simulink model "vMCU_model"  (R2024b)
settings: Solver=FixedStepAuto  StartTime=0.0  StopTime=0.15  FixedStep=125e-9  RelTol=1e-3
undefined symbols (not defined in the file): den, num
settings Model: Creator=matti  LastModifiedBy=Andrei
settings SolverCC: AlgebraicLoopSolver=TrustRegion
settings DebuggingCC: UnconnectedInputMsg=warning  UnconnectedOutputMsg=warning  UnconnectedLineMsg=warning
settings ModelReferenceCC: EnableRefExpFcnMdlSchedulingChecks=on
settings RTWCC: GPUComputeCapability=3.5

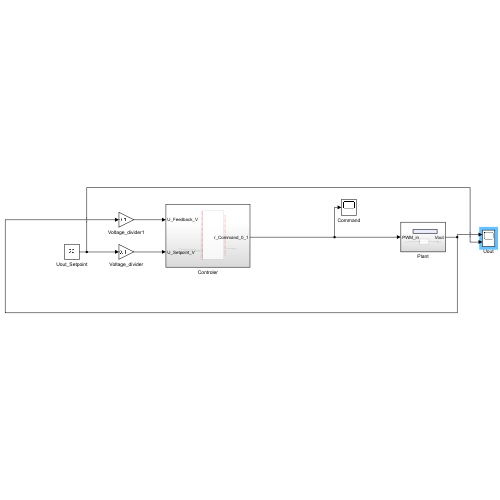
[thumbnail: Simulink's stored preview of the top-level diagram]
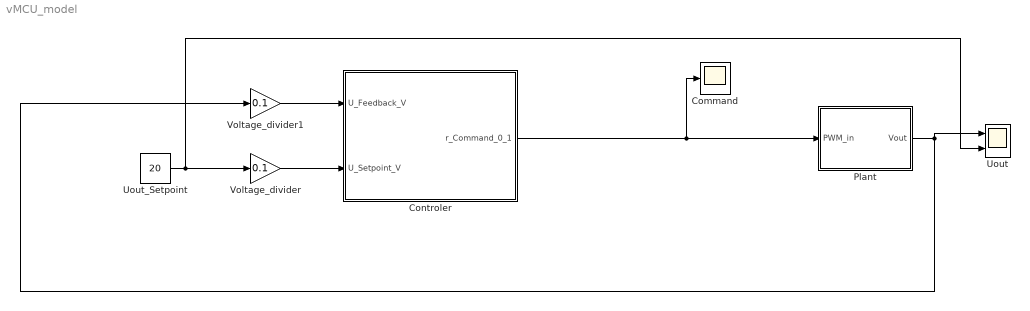
== system vMCU_model ==
  Command : Scope
  Controler : Subsystem
  Plant : Subsystem
  Uout : Scope  NumInputPorts=2
  Uout_Setpoint : Constant  Value=20
  Voltage_divider : Gain  Gain=0.1
  Voltage_divider1 : Gain  Gain=0.1
  wires:
  Voltage_divider1/1 -> Controler/1(U_Feedback_V)
  Uout_Setpoint/1 -> Uout/2, Voltage_divider/1
  Controler/1(r_Command_0_1) -> Plant/1(PWM_in), Command/1
  Plant/1(Vout) -> Voltage_divider1/1, Uout/1
  Voltage_divider/1 -> Controler/2(U_Setpoint_V)

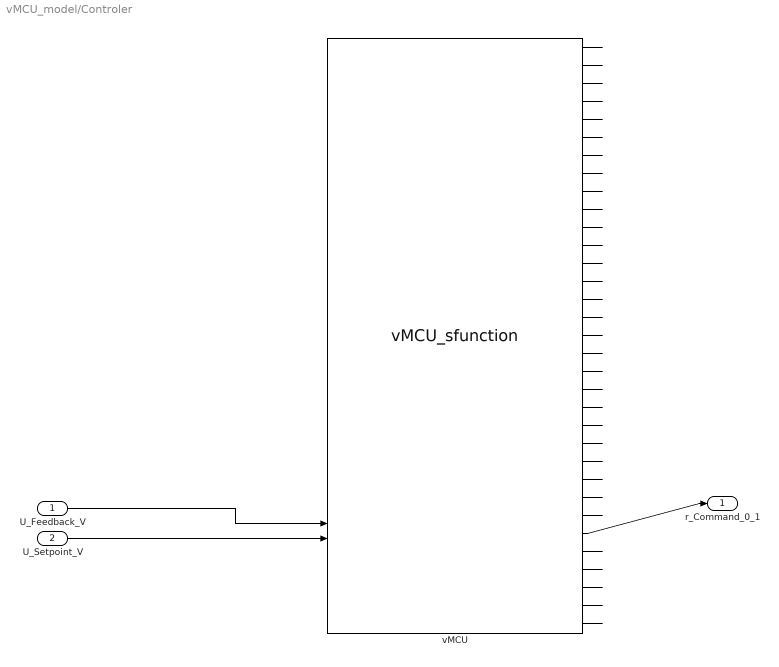
== system vMCU_model/Controler ==
  U_Feedback_V : Inport
  U_Setpoint_V : Inport  Port=2
  vMCU : S-Function  FunctionName=vMCU_sfunction  SFunctionDeploymentMode=off  EnableBusSupport=off
      mask Display:
      | port_label('output', 1, 'vPA0_O_D')
      | port_label('output', 2, 'vPA1_O_D')
      | port_label('output', 3, 'vPA2_O_D')
      | port_label('output', 4, 'vPA3_O_D')
      | port_label('output', 5, 'vPA4_O_D')
      | port_label('output', 6, 'vPA5_O_D')
      | port_label('output', 7, 'vPA6_O_D')
      | port_label('output', 8, 'vPA7_O_D')
      | port_label('output', 9, 'vPB0_O_D')
      | port_label('output', 10, 'vPB1_O_D')
      | port_label('output', 11, 'vPB2_O_D')
      | port_label('output', 12, 'vPB3_O_D')
      | port_label('output', 13, 'vPB4_O_D')
      | port_label('output', 14, 'vPB5_O_D')
      | port_label('output', 15, 'vPB6_O_D')
      | port_label('output', 16, 'vPB7_O_D')
      | port_label('output', 17, 'vPC0_O_D')
      | port_label('output', 18, 'vPC1_O_D')
      | port_label('output', 19, 'vPC2_O_D')
      | port_label('output', 20, 'vPC3_O_D')
      | port_label('output', 21, 'vPC4_O_D')
      | port_label('output', 22, 'vPC5_O_D')
      | port_label('output', 23, 'vPC6_O_D')
      | port_label('output', 24, 'vPC7_O_D')
      | port_label('output', 25, 'vPD0_O_D')
      | port_label('output', 26, 'vPD1_O_D')
      | port_label('output', 27, 'vPD2_O_D')
      | port_label('output', 28, 'vPD3_O_D')
      | port_label('output', 29, 'vPD4_O_D')
      | port_label('output', 30, 'vPD5_O_D')
      | port_label('output', 31, 'vPD6_O_D')
      | port_label('output', 32, 'vPD7_O_D')
      | port_label('output', 33, 'DEBUG_port')
      | 
      | port_label('input', 1, 'vPA0_I_D')
      | port_label('input', 2, 'vPA1_I_D')
      | port_label('input', 3, 'vPA2_I_D')
      | port_label('input', 4, 'vPA3_I_D')
      | port_label('input', 5, 'vPA4_I_D')
      | port_label('input', 6, 'vPA5_I_D')
      | port_label('input', 7, 'vPA6_I_D')
      | port_label('input', 8, 'vPA7_I_D')
      | port_label('input', 9, 'vPB0_I_D')
      | port_label('input', 10, 'vPB1_I_D')
      | port_label('input', 11, 'vPB2_I_D')
      | port_label('input', 12, 'vPB3_I_D')
      | port_label('input', 13, 'vPB4_I_D')
      | port_label('input', 14, 'vPB5_I_D')
      | port_label('input', 15, 'vPB6_I_D')
      | port_label('input', 16, 'vPB7_I_D')
      | port_label('input', 17, 'vPC0_I_D')
      | port_label('input', 18, 'vPC1_I_D')
      | port_label('input', 19, 'vPC2_I_D')
      | port_label('input', 20, 'vPC3_I_D')
      | port_label('input', 21, 'vPC4_I_D')
      | port_label('input', 22, 'vPC5_I_D')
      | port_label('input', 23, 'vPC6_I_D')
      | port_label('input', 24, 'vPC7_I_D')
      | port_label('input', 25, 'vPD0_I_D')
      | port_label('input', 26, 'vPD1_I_D')
      | port_label('input', 27, 'vPD2_I_D')
      | port_label('input', 28, 'vPD3_I_D')
      | port_label('input', 29, 'vPD4_I_D')
      | port_label('input', 30, 'vPD5_I_D')
      | port_label('input', 31, 'vPD6_I_D')
      | port_label('input', 32, 'vPD7_I_D')
      | port_label('input', 33, 'vPA0_I_A')
      | port_label('input', 34, 'vPA1_I_A')
      | port_label('input', 35, 'vPA2_I_A')
      | port_label('input', 36, 'vPA3_I_A')
      | port_label('input', 37, 'vPA4_I_A')
      | port_label('input', 38, 'vPA5_I_A')
      | port_label('input', 39, 'vPA6_I_A')
      | port_label('input', 40, 'vPA7_I_A')
  r_Command_0_1 : Outport
  wires:
  vMCU/18 -> ?
  ? -> vMCU/5
  vMCU/16 -> ?
  ? -> vMCU/16
  U_Feedback_V/1 -> vMCU/33
  ? -> vMCU/19
  vMCU/28 -> r_Command_0_1/1
  ? -> vMCU/20
  ? -> vMCU/1
  U_Setpoint_V/1 -> vMCU/34
  vMCU/10 -> ?
  ? -> vMCU/21
  ? -> vMCU/38
  vMCU/5 -> ?
  ? -> vMCU/40
  ? -> vMCU/11
  ? -> vMCU/3
  ? -> vMCU/25
  vMCU/11 -> ?
  vMCU/20 -> ?
  ? -> vMCU/4
  ? -> vMCU/6
  ? -> vMCU/2
  ? -> vMCU/7
  ? -> vMCU/10
  ? -> vMCU/35
  vMCU/22 -> ?
  ? -> vMCU/9
  vMCU/4 -> ?
  ? -> vMCU/27
  vMCU/7 -> ?
  ? -> vMCU/36
  ? -> vMCU/8
  vMCU/25 -> ?
  ? -> vMCU/15
  ? -> vMCU/14
  ? -> vMCU/37
  ? -> vMCU/13
  ? -> vMCU/12
  ? -> vMCU/31
  ? -> vMCU/18
  vMCU/30 -> ?
  vMCU/19 -> ?
  vMCU/14 -> ?
  vMCU/6 -> ?
  ? -> vMCU/17
  ? -> vMCU/22
  ? -> vMCU/23
  ? -> vMCU/24
  vMCU/17 -> ?
  ? -> vMCU/32
  ? -> vMCU/30
  ? -> vMCU/26
  vMCU/13 -> ?
  ? -> vMCU/29
  vMCU/12 -> ?
  ? -> vMCU/28
  vMCU/15 -> ?
  ? -> vMCU/39
  vMCU/3 -> ?
  vMCU/1 -> ?
  vMCU/2 -> ?
  vMCU/24 -> ?
  vMCU/9 -> ?
  vMCU/8 -> ?
  vMCU/23 -> ?
  vMCU/21 -> ?
  vMCU/31 -> ?
  vMCU/29 -> ?
  vMCU/26 -> ?
  vMCU/27 -> ?
  vMCU/32 -> ?
  vMCU/33 -> ?

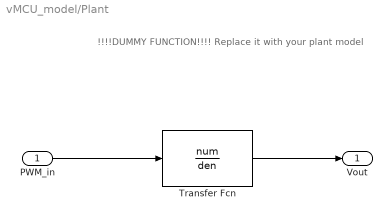
== system vMCU_model/Plant ==
  note: !!!!DUMMY FUNCTION!!!!
      | Replace it with your plant model
  PWM_in : Inport
  Transfer Fcn : TransferFcn  Numerator=num  Denominator=den
  Vout : Outport
  wires:
  Transfer Fcn/1 -> Vout/1
  PWM_in/1 -> Transfer Fcn/1
